simulink model "ImpulseSDOF_2Pedestrian_sim"  (R2022a)
settings: Solver=ode4  StartTime=t_inicial  StopTime=t_final  FixedStep=t_step  RelTol=1e-3
values from neighbouring files (symbols this model uses):
  A = [0 1; -w^2 -2*xi*w]    [Bridge_3Pedestrians.m]
  ai = 1    [Bridge_3Pedestrians.m]
  ai2 = 0.5    [Bridge_3Pedestrians.m]
  ai3 = 0.01    [Bridge_3Pedestrians.m]
  B = [0; 1/Mspan]    [Bridge_3Pedestrians.m]
  C = [1 0; 0 1; -w^2 -2*xi*w]    [Bridge_3Pedestrians.m]
  D = [0;0; 1/Mspan]    [Bridge_3Pedestrians.m]
  lambdai = 0.6    [Bridge_3Pedestrians.m]
  lambdai2 = 0.5    [Bridge_3Pedestrians.m]
  lambdai3 = 0.3    [Bridge_3Pedestrians.m]
  mi = 70    [Bridge_3Pedestrians.m]
  mi2 = 75    [Bridge_3Pedestrians.m]
  wi = 2*pi*fi    (= 5.3407075111)    [Bridge_3Pedestrians.m]
  wi2 = 2*pi*fi    (= 5.3407075111)    [Bridge_3Pedestrians.m]
  wi3 = 2*pi*fi    (= 5.3407075111)    [Bridge_3Pedestrians.m]
libraries: cstblocks x1
settings Model: Creator=Javiera  LastModifiedBy=LEGION
settings DebuggingCC: AlgebraicLoopMsg=none  UnconnectedInputMsg=warning  UnconnectedOutputMsg=warning  UnconnectedLineMsg=warning  SFMachineParentedDataDiag=warning

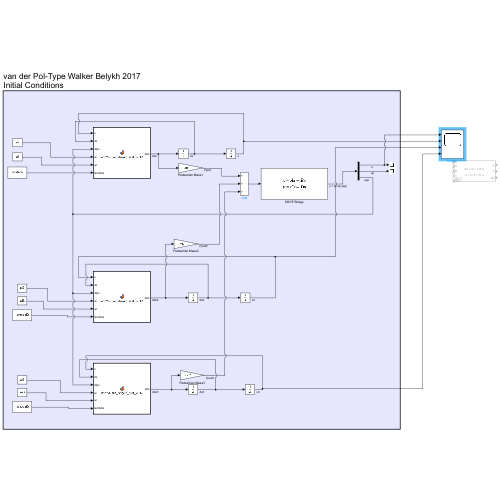
[thumbnail: Simulink's stored preview of the top-level diagram]
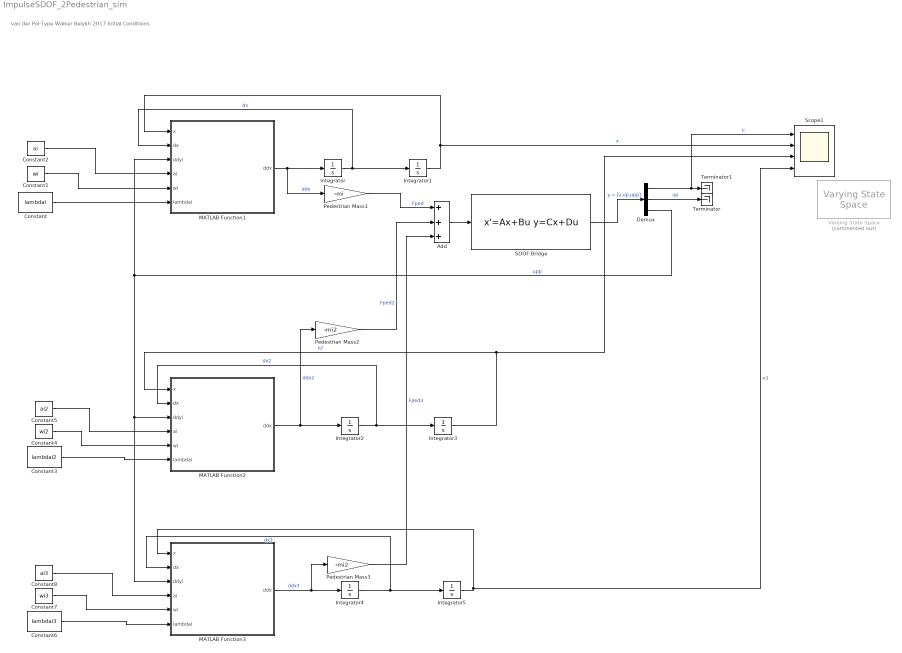
== system ImpulseSDOF_2Pedestrian_sim ==
  note: van der Pol-Type Walker Belykh 2017
      | Initial Conditions
  Add : Sum  Inputs=+++
  Constant : Constant  Value=lambdai
  Constant1 : Constant  Value=wi
  Constant2 : Constant  Value=ai
  Constant3 : Constant  Value=lambdai2
  Constant4 : Constant  Value=wi2
  Constant5 : Constant  Value=ai2
  Constant6 : Constant  Value=lambdai3
  Constant7 : Constant  Value=wi3
  Constant8 : Constant  Value=ai3
  Demux : Demux  Outputs=3
  Integrator : Integrator
  Integrator1 : Integrator  InitialCondition=-0.02
  Integrator2 : Integrator
  Integrator3 : Integrator  InitialCondition=0.05
  Integrator4 : Integrator
  Integrator5 : Integrator  InitialCondition=0.03
  MATLAB Function1 : MATLAB Function  TreatAsAtomicUnit=on
  MATLAB Function2 : MATLAB Function  TreatAsAtomicUnit=on
  MATLAB Function3 : MATLAB Function  TreatAsAtomicUnit=on
  Pedestrian Mass1 : Gain  Gain=-mi
  Pedestrian Mass2 : Gain  Gain=-mi2
  Pedestrian Mass3 : Gain  Gain=-mi2
  SDOF Bridge : StateSpace  A=A  B=B  C=C  D=D  InitialCondition=[0.05;0]
  Scope1 : Scope  NumInputPorts=4
  Terminator : Terminator
  Terminator1 : Terminator
  Varying State Space : cstblocks/Linear Parameter Varying/Varying State Space  Commented=on  x0=0  xNames=''  OutputX=on  OutputDX=on
  wires:
  MATLAB Function1/1(ddx) -> Integrator/1, Pedestrian Mass1/1  "ddx"
  Integrator/1 -> MATLAB Function1/2(dx), Integrator1/1  "dx"
  Integrator1/1 -> Scope1/2, MATLAB Function1/1(x)  "x"
  Demux/3 -> MATLAB Function1/3(ddyi), MATLAB Function3/3(ddyi), MATLAB Function2/3(ddyi)  "upp"
  Demux/2 -> Terminator/1  "up"
  Demux/1 -> Scope1/1, Terminator1/1  "u"
  Constant2/1 -> MATLAB Function1/4(ai)
  Constant1/1 -> MATLAB Function1/5(wi)
  Constant/1 -> MATLAB Function1/6(lambdai)
  MATLAB Function2/1(ddx) -> Integrator2/1, Pedestrian Mass2/1  "ddx2"
  Constant3/1 -> MATLAB Function2/6(lambdai)
  Constant5/1 -> MATLAB Function2/4(ai)
  Constant4/1 -> MATLAB Function2/5(wi)
  Integrator2/1 -> MATLAB Function2/2(dx), Integrator3/1  "dx2"
  Integrator3/1 -> MATLAB Function2/1(x), Scope1/3  "x2"
  Pedestrian Mass2/1 -> Add/2  "Fped2"
  Pedestrian Mass1/1 -> Add/1  "Fped"
  Add/1 -> SDOF Bridge/1
  SDOF Bridge/1 -> Demux/1  "y = [u,up,upp]"
  Constant8/1 -> MATLAB Function3/4(ai)
  Constant7/1 -> MATLAB Function3/5(wi)
  Constant6/1 -> MATLAB Function3/6(lambdai)
  MATLAB Function3/1(ddx) -> Pedestrian Mass3/1, Integrator4/1  "ddx3"
  Integrator4/1 -> MATLAB Function3/2(dx), Integrator5/1  "dx3"
  Integrator5/1 -> Scope1/4, MATLAB Function3/1(x)  "x3"
  Pedestrian Mass3/1 -> Add/3  "Fped3"

== matlab function ImpulseSDOF_2Pedestrian_sim/MATLAB Function1 ==
  data: x input; ddx output; dx input; ddyi input; ai input; wi input; lambdai input
function ddx = vdpWalker_Belykh_etal_2017(x,dx,ddyi,ai,wi,lambdai)
% Alexis Contreras R. 

% Foot force models of crowd dynamics on a wobbly bridge
% Igor V. Belykh, Russel Jeter and Vladimir N. Belykh (2017)

% Modelo de peatón de oscilador auto-sostenible donde los pasos se ajustan
% al movimiento del puente. El balance humano se modela como péndulo invertido.
% de la forma de oscilador van der Pol (vdP)

% Inputs:
% x         -> Desplazamiento del centro de masa (CoM) del peatón
% dx        -> Velocidad del centro de masa del peatón 
% ddyi      -> Aceleración absoluta del puente (o relativa al suelo/punto fijo externo)
% lambdai   -> Parámetro de amortiguamiento
% ai        -> Parámetro de control del mecanismo de auto-excitación del caminar humano
% wi        -> wi = sqrt(g/L), del modelo pendulo invertido (L >> x)

% Outputs:
% ddx       -> Aceleración del peatón

fxdx = lambdai*(dx^2 + x^2 - ai^2)*dx + wi^2*x;                              % (Eq.5)
ddx = -ddyi - fxdx;                                                         % (Eq.1)

== matlab function ImpulseSDOF_2Pedestrian_sim/MATLAB Function2 ==
  data: x input; ddx output; dx input; ddyi input; ai input; wi input; lambdai input
function ddx = vdpWalker_Belykh_etal_2017(x,dx,ddyi,ai,wi,lambdai)
% Alexis Contreras R. 

% Foot force models of crowd dynamics on a wobbly bridge
% Igor V. Belykh, Russel Jeter and Vladimir N. Belykh (2017)

% Modelo de peatón de oscilador auto-sostenible donde los pasos se ajustan
% al movimiento del puente. El balance humano se modela como péndulo invertido.
% de la forma de oscilador van der Pol (vdP)

% Inputs:
% x         -> Desplazamiento del centro de masa (CoM) del peatón
% dx        -> Velocidad del centro de masa del peatón 
% ddyi      -> Aceleración absoluta del puente (o relativa al suelo/punto fijo externo)
% lambdai   -> Parámetro de amortiguamiento
% ai        -> Parámetro de control del mecanismo de auto-excitación del caminar humano
% wi        -> wi = sqrt(g/L), del modelo pendulo invertido (L >> x)

% Outputs:
% ddx       -> Aceleración del peatón

fxdx = lambdai*(dx^2 + x^2 - ai^2)*dx + wi^2*x;                              % (Eq.5)
ddx = -ddyi - fxdx;                                                         % (Eq.1)

== matlab function ImpulseSDOF_2Pedestrian_sim/MATLAB Function3 ==
  data: x input; ddx output; dx input; ddyi input; ai input; wi input; lambdai input
function ddx = vdpWalker_Belykh_etal_2017(x,dx,ddyi,ai,wi,lambdai)
% Alexis Contreras R. 

% Foot force models of crowd dynamics on a wobbly bridge
% Igor V. Belykh, Russel Jeter and Vladimir N. Belykh (2017)

% Modelo de peatón de oscilador auto-sostenible donde los pasos se ajustan
% al movimiento del puente. El balance humano se modela como péndulo invertido.
% de la forma de oscilador van der Pol (vdP)

% Inputs:
% x         -> Desplazamiento del centro de masa (CoM) del peatón
% dx        -> Velocidad del centro de masa del peatón 
% ddyi      -> Aceleración absoluta del puente (o relativa al suelo/punto fijo externo)
% lambdai   -> Parámetro de amortiguamiento
% ai        -> Parámetro de control del mecanismo de auto-excitación del caminar humano
% wi        -> wi = sqrt(g/L), del modelo pendulo invertido (L >> x)

% Outputs:
% ddx       -> Aceleración del peatón

fxdx = lambdai*(dx^2 + x^2 - ai^2)*dx + wi^2*x;                              % (Eq.5)
ddx = -ddyi - fxdx;                                                         % (Eq.1)
